simulink model "rtwdemo_cppencap_refbot"  (Simulink 7.6)
settings: Solver=FixedStepDiscrete  SolverMode=SingleTasking  StartTime=0.0  StopTime=100.0  FixedStep=0.1  RelTol=1e-3
libraries: rtwdemowidgets x1
Description:
  | Example model reference component.
settings Model: Creator=The MathWorks Inc.  ExtModeAutoUpdateStatusClock=off
settings DataIOCC: SaveOutput=off  SignalLogging=off  SaveTime=off  SignalLoggingName=sigsOut
settings OptimizationCC: InlineParams=on  InlineInvariantSignals=on  StateBitsets=on  DataBitsets=on  UseTempVars=on  ZeroExternalMemoryAtStartup=off  NoFixptDivByZeroProtection=on  EfficientFloat2IntCast=on  EfficientMapNaN2IntZero=off  OptimizeModelRefInitCode=on  LifeSpan=1
settings DebuggingCC: SignalInfNanChecking=error  AlgebraicLoopMsg=error  ArtificialAlgebraicLoopMsg=error  UnderspecifiedInitializationDetection=Simplified  MergeDetectMultiDrivingBlocksExec=error  CheckExecutionContextPreStartOutputMsg=on  CheckExecutionContextRuntimeOutputMsg=on  BlockPriorityViolationMsg=error  MinStepSizeMsg=error  SolverPrmCheckMsg=error  InheritedTsInSrcMsg=error  DiscreteInheritContinuousMsg=error  SingleTaskRateTransMsg=error  TasksWithSamePriorityMsg=error  SigSpecEnsureSampleTimeMsg=error  CheckMatrixSingularityMsg=error  IntegerOverflowMsg=error  ParameterUnderflowMsg=error  ParameterPrecisionLossMsg=error  ParameterTunabilityLossMsg=error  UnderSpecifiedDataTypeMsg=error  UniqueDataStoreMsg=error  UnknownTsInhSupMsg=error  StrictBusMsg=ErrorOnBusTreatedAsVector
settings HardwareCC: ProdIntDivRoundTo=Zero  ProdEndianess=LittleEndian  ProdHWDeviceType=Generic->32-bit Embedded Processor  TargetHWDeviceType=Generic->32-bit Embedded Processor
settings RTWCC: SystemTargetFile=ert.tlc  TLCOptions=-p0  TemplateMakefile=ert_default_tmf  Description=Real-Time Workshop Embedded Coder (no auto configuration)  GenerateReport=on  RTWVerbose=off  ProcessScript=ert_make_rtw_hook  IncludeHyperlinkInReport=on  LaunchReport=on  TargetLang=C++ (Encapsulated)  GenerateTraceInfo=on  GenerateTraceReport=on  GenerateTraceReportSl=on  GenerateTraceReportSf=on  GenerateTraceReportEml=on
settings CodeAppCC: ForceParamTrailComments=on  IgnoreTestpoints=on  MaxIdLength=128  SimulinkDataObjDesc=on  CustomSymbolStrGlobalVar=rt$N$M  CustomSymbolStrType=$N$M  CustomSymbolStrFcn=$N$M$F  CustomSymbolStrMacro=$N$M  InsertBlockDesc=on
settings ERTTargetCC: MultiwordLength=2048  GenerateSampleERTMain=on  IncludeMdlTerminateFcn=off  MultiInstanceERTCode=on  SupportNonFinite=off  SupportComplex=off  InlinedParameterPlacement=NonHierarchical  RootIOFormat=Structure reference  ERTCustomFileTemplate=example_file_process.tlc  ConvertIfToSwitch=off
settings ERTCPPComponent: GenerateDestructor=on  GenerateExternalIOAccessMethods=None  ParameterMemberVisibility=private  InternalMemberVisibility=private  GenerateParameterAccessMethods=None  GenerateInternalMemberAccessMethods=None  UseOperatorNewForModelRefRegistration=off

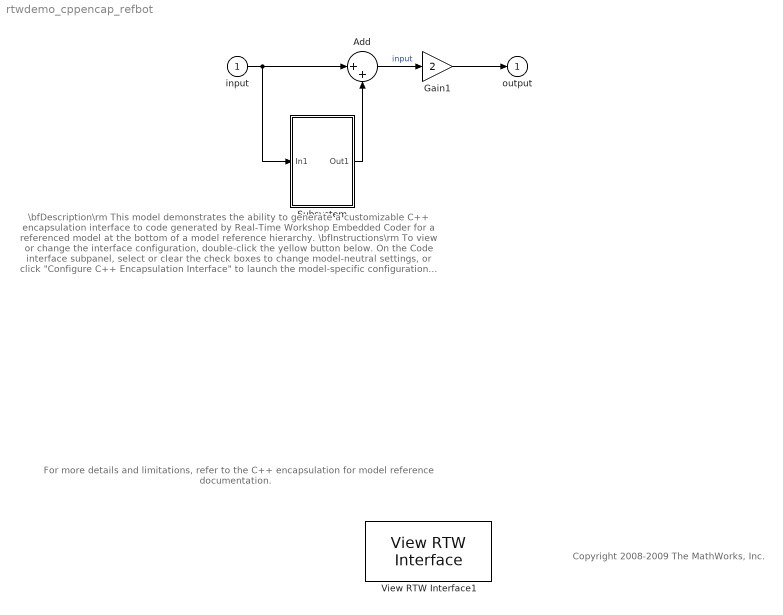
== system rtwdemo_cppencap_refbot ==
  note: Copyright 2008-2009 The MathWorks, Inc.
  note: \bfDescription\rm
      | This model demonstrates the ability to generate a customizable C++ encapsulation interface to
      | code generated by Real-Time Workshop Embedded Coder for a referenced model at the bottom of
      | a model reference hierarchy.
      | \bfInstructions\rm
      |    To view or change the interface configuration, double-click the yellow button below. On the Code
      |    interface subpanel, select or clear the check boxes to change model-neutral settings, or click
      |    "Configure C++ Encapsulation Interface" to launch the model-specific configuration dialog box.
      |
      | To configure a new or existing referenced model for C++ encapsulation, choose "ert.tlc" as the system
      | target file on the Real-Time Workshop page, and then set the Language to "C++ (Encapsulated)".
      | Go to the Interface page to configure the C++ encapsulation interface for the model. In the dialog
      | box launched by the "Configure C++ Encapsulation Interface" button, make sure
      | "I/O arguments step method" is selected for the Function specification.
  note: For more details and limitations, refer to the C++ encapsulation for model reference documentation.
  " input" : Inport  OutDataTypeStr=double  PortDimensions=1  SampleTime=0.1
  Add : Sum  Inputs=|++
  Gain1 : Gain  Gain=2
  Subsystem : Subsystem  TreatAsAtomicUnit=on
  View RTW Interface1 : rtwdemowidgets/View RTW Interface  SystemSampleTime=-1
  output : Outport
  wires:
  " input"/1 -> Add/1, Subsystem/1(In1)
  Add/1 -> Gain1/1  "input"
  Gain1/1 -> output/1
  Subsystem/1(Out1) -> Add/2

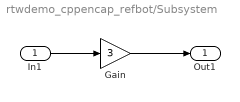
== system rtwdemo_cppencap_refbot/Subsystem ==
  In1 : Inport
  Gain : Gain  Gain=3
  Out1 : Outport
  wires:
  Gain/1 -> Out1/1
  In1/1 -> Gain/1
